simulink model "threephasefullconverter"  (R2013b)
settings: Solver=ode45  StartTime=0.0  StopTime=0.04  RelTol=1e-3
undefined symbols (not defined in the file): alpha
libraries: powerlib x13
settings Model: Creator=SAI KUMAR  LastModifiedBy=SAI KUMAR

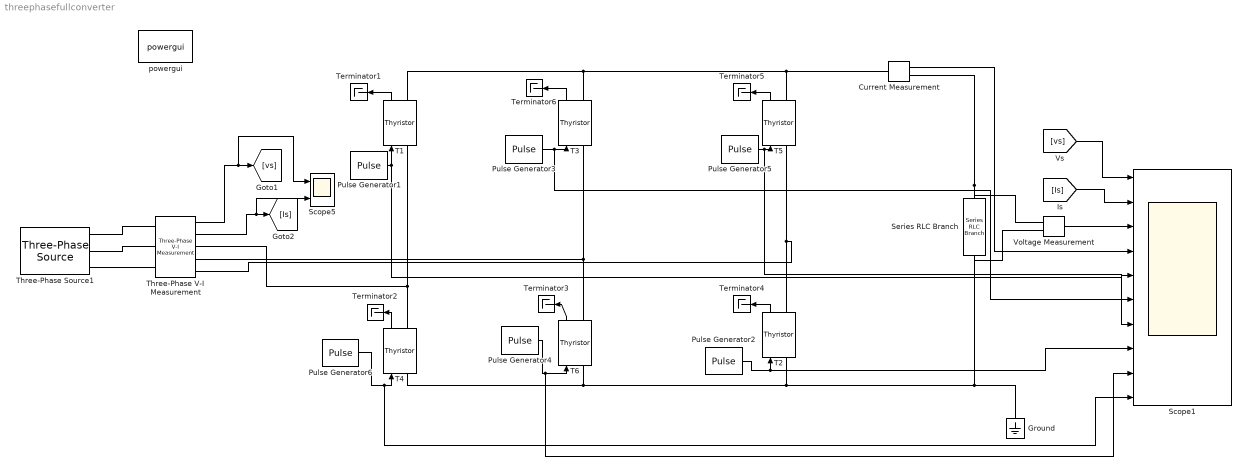
== system threephasefullconverter ==
  Current Measurement : powerlib/Measurements/Current Measurement  PhasorSimulation=off  OutputType=Complex  PSBequivalent=0
  Ground : powerlib/Elements/Ground  LConnTagsString=a
  Pulse Generator1 : DiscretePulseGenerator  PulseType=Time based  Amplitude=5  Period=0.02  PulseWidth=10  PhaseDelay=((0.02/360)*alpha)+((0.02/360)*30)
  Pulse Generator2 : DiscretePulseGenerator  PulseType=Time based  Amplitude=5  Period=0.02  PulseWidth=10  PhaseDelay=((0.02/360)*alpha)+((0.02/360)*90)
  Pulse Generator3 : DiscretePulseGenerator  PulseType=Time based  Amplitude=5  Period=0.02  PulseWidth=10  PhaseDelay=((0.02/360)*alpha)+((0.02/360)*150)
  Pulse Generator4 : DiscretePulseGenerator  PulseType=Time based  Amplitude=5  Period=0.02  PulseWidth=10  PhaseDelay=((0.02/360)*alpha)+((0.02/360)*330)
  Pulse Generator5 : DiscretePulseGenerator  PulseType=Time based  Amplitude=5  Period=0.02  PulseWidth=10  PhaseDelay=((0.02/360)*alpha)+((0.02/360)*270)
  Pulse Generator6 : DiscretePulseGenerator  PulseType=Time based  Amplitude=5  Period=0.02  PulseWidth=10  PhaseDelay=((0.02/360)*alpha)+((0.02/360)*210)
  Scope1 : Scope  NumInputPorts=10
      settings: TimeRange=5  YMin=5~-5~-5~-5~-5~-5~-5~-5~-5~-5  YMax=85~5~5~5~5~5~5~5~5~5  SampleInput=on
  Scope5 : Scope  NumInputPorts=2
      settings: TimeRange=5  YMin=5~-5  YMax=85~5  SampleInput=on
  Series RLC Branch : powerlib/Elements/Series RLC Branch  LConnTagsString=__new0  RConnTagsString=__new0  BranchType=R  Resistance=10  Inductance=1e-3  SetiL0=off  InitialCurrent=0  Capacitance=1e-6  Setx0=off  InitialVoltage=0  Measurements=None
  T{1..6} (6 alike) : powerlib/Power Electronics/Thyristor  Ron=0.001  Lon=0  Vf=0.8  IC=0  Rs=500  Cs=250e-9  Measurements=on
  Terminator{1..6} (6 alike) : Terminator
  Three-Phase V-I Measurement : powerlib/Measurements/Three-Phase V-I Measurement  VoltageMeasurement=phase-to-phase  SetLabelV=off  LabelV=Vabc  Vpu=off  VpuLL=off  CurrentMeasurement=yes  SetLabelI=off  LabelI=Iabc  Ipu=off  Pbase=100e6  Vbase=500e3  OutputType=Complex  PhasorSimulation=off  PSBequivalent=0
  Three-Phase Source1 : powerlib/Electrical Sources/Three-Phase Source  Voltage=25e3  PhaseAngle=0  Frequency=50  InternalConnection=Yg  SpecifyImpedance=off  Resistance=0.8929  Inductance=16.58e-3  ShortCircuitLevel=100e6  BaseVoltage=25e3  XRratio=7  BusType=swing  Pref=0  Qref=0  Qmin=-inf  Qmax=inf
  Voltage Measurement : powerlib/Measurements/Voltage Measurement  PhasorSimulation=off  OutputType=Complex  PSBequivalent=0
  powergui : powerlib/powergui  Priority=1  SimulationMode=Continuous  SolverType=Tustin  SampleTime=50e-6  frequency=60  SPID=off  DisableSnubberDevices=off  DisableRonSwitches=off  DisableVfSwitches=off  SwTol=0  Interpol=off  DisplayEquations=off  frequencyindice=0  Pbase=100e6  ErrMax=1e-4  Iterations=50  UnitsV=kV  UnitsW=MW  FunctionMessages=off  echomessages=off  HookPort=off  EnableUseOfTLC=off  x0status=blocks  RestoreLinks=warning  ResistiveCurrentMeasurement=off  Frange=[0:2:500]  Ylog=off  Xlog=on  ShowGrid=off  save=off  variable=ZData  ZoomFFT=off  StartTime=0.0  cycles=1  DisplayStyle=1  fundamental=60  FreqAxis=off  MaxFrequency=1000  frequencyindicesteady=1  RmsSteady=1  display=off  Ts=0  methode=off
  wires:
  Pulse Generator1/1 -> T1/1, Scope1/5
  Pulse Generator2/1 -> Scope1/8, T2/1
  Pulse Generator4/1 -> Scope1/9, T6/1
  Pulse Generator6/1 -> Scope1/10, T4/1
  T1/1 -> Terminator1/1
  T4/1 -> Terminator2/1
  T6/1 -> Terminator3/1
  T5/1 -> Terminator5/1
  T3/1 -> Terminator6/1
  Voltage Measurement/1 -> Scope1/3
  Current Measurement/1 -> Scope1/4
  [vs] -> Scope1/1
  [Is] -> Scope1/2
  Pulse Generator3/1 -> Scope1/6, T3/1
  Pulse Generator5/1 -> Scope1/7, T5/1
  Three-Phase V-I Measurement/1 -> Scope5/1, [vs]
  Three-Phase V-I Measurement/2 -> Scope5/2, [Is]
  T2/1 -> Terminator4/1
  connections:
  T1/LConn1 -- Three-Phase V-I Measurement/RConn1 -- T4/RConn1
  T3/LConn1 -- Three-Phase V-I Measurement/RConn2 -- T6/RConn1
  T5/LConn1 -- T2/RConn1 -- Three-Phase V-I Measurement/RConn3
  T1/RConn1 -- T3/RConn1 -- Current Measurement/LConn1 -- T5/RConn1
  T4/LConn1 -- T6/LConn1 -- Ground/LConn1 -- Voltage Measurement/LConn2 -- Series RLC Branch/RConn1 -- T2/LConn1
  Current Measurement/RConn1 -- Voltage Measurement/LConn1 -- Series RLC Branch/LConn1
  Three-Phase Source1/RConn1 -- Three-Phase V-I Measurement/LConn1
  Three-Phase Source1/RConn2 -- Three-Phase V-I Measurement/LConn2
  Three-Phase Source1/RConn3 -- Three-Phase V-I Measurement/LConn3
